simulink model "RNDBitGen"  (R2014b)
settings: Solver=FixedStepDiscrete  SolverMode=SingleTasking  StartTime=0.0  StopTime=20e-6*2  RelTol=1e-3
PreLoadFcn:
  | userName = getenv('UserName');
  | 
  | if strcmp(userName,'Tim')
  | cd C:\MA_1\RNDBitGen
  | else
  | cd D:\MA_1\RNDBitGen
  | end
InitFcn:
  | userName = getenv('UserName');
  | 
  | if strcmp(userName,'Tim')
  | cd C:\MA_1\RNDBitGen
  | else
  | cd D:\MA_1\RNDBitGen
  | end
libraries: xbsIndex_r4 x30
settings Model: Creator=Tim-UML  LastModifiedBy=Tim-UML
settings DebuggingCC: AssertControl=DisableAll
settings HardwareCC: ProdBitPerLong=64  ProdBitPerPointer=64  ProdWordSize=64  ProdHWDeviceType=Generic->64-bit Embedded Processor (LP64)  TargetHWDeviceType=32-bit Generic

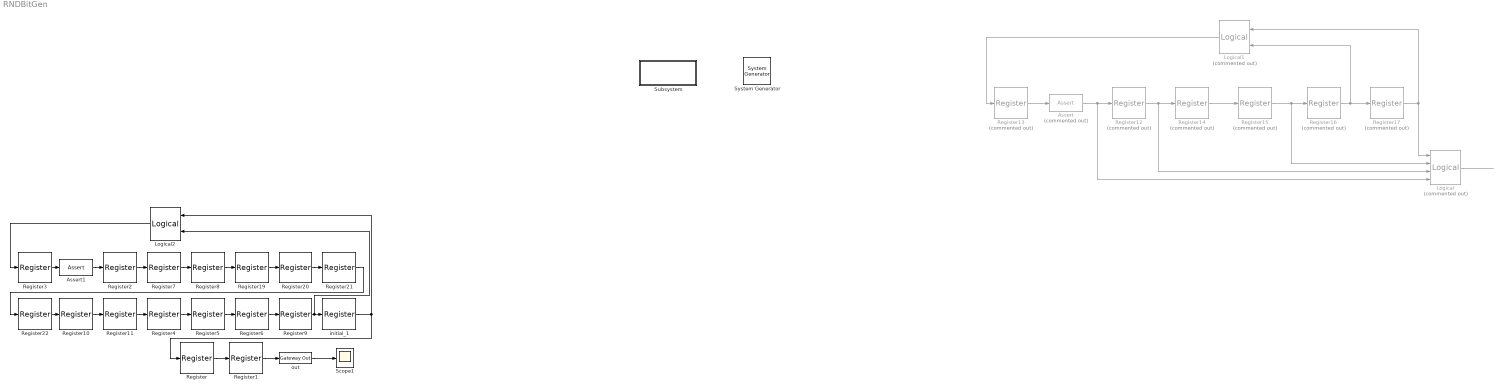
== system RNDBitGen ==
  " System Generator" : xbsIndex_r4/ System Generator  Tag=genX  xilinxfamily=zynq  part=xc7z020  speed=-1  package=clg400  synthesis_tool=Vivado  clock_wrapper=Clock Enables  directory=./netlistFin1  proj_type=Vivado  Synth_file=Vivado Synthesis Defaults  Impl_file=Vivado Implementation Defaults  testbench=on  simulink_period=sysgenSystemPeriod  sysclk_period=1000/250  dcm_input_clock_period=10  incr_netlist=off  trim_vbits=Everywhere in SubSystem  dbl_ovrd=According to Block Masks  core_generation=According to Block Masks  run_coregen=off  deprecated_control=off  eval_field=0  block_type=sysgen
  Assert : xbsIndex_r4/Assert  Commented=on  assert_type=on  type_source=Explicitly  gui_display_data_type=Boolean  arith_type=Boolean  n_bits=16  bin_pt=14  preci_type=Single  exp_width=8  frac_width=24  assert_rate=on  rate_source=Explicitly  period=Tb  output_port=on  block_type=assert
  Assert1 : xbsIndex_r4/Assert  assert_type=on  type_source=Explicitly  gui_display_data_type=Boolean  arith_type=Boolean  n_bits=16  bin_pt=14  preci_type=Single  exp_width=8  frac_width=24  assert_rate=on  rate_source=Explicitly  period=Tb  output_port=on  block_type=assert
  Logical : xbsIndex_r4/Logical  Commented=on  logical_function=XOR  inputs=4  en=off  latency=0  precision=Full  arith_type=Unsigned  n_bits=16  bin_pt=0  align_bp=on  dbl_ovrd=off  block_type=logical
  Logical1 : xbsIndex_r4/Logical  Commented=on  logical_function=XOR  inputs=2  en=off  latency=0  precision=Full  arith_type=Unsigned  n_bits=16  bin_pt=0  align_bp=on  dbl_ovrd=off  block_type=logical
  Logical2 : xbsIndex_r4/Logical  logical_function=XOR  inputs=2  en=off  latency=0  precision=Full  arith_type=Unsigned  n_bits=16  bin_pt=0  align_bp=on  dbl_ovrd=off  block_type=logical
  Register{,1..11,19..22} (16 alike) : xbsIndex_r4/Register  init=0  rst=off  en=off  dbl_ovrd=off  block_type=register
  Register{12..16} (5 alike) : xbsIndex_r4/Register  Commented=on  init=0  rst=off  en=off  dbl_ovrd=off  block_type=register
  Register17 : xbsIndex_r4/Register  Commented=on  init=1  rst=off  en=off  dbl_ovrd=off  block_type=register
  Scope1 : Scope
      settings: TimeRange=1.102458307597285e-07  YMin=-0  YMax=2  SaveName=ScopeData92
  Subsystem : Subsystem  mask(Model Parameters){upsample=No, dmtOfdm=DMT, guardInterval=Yes, AWGN=No, channel=No, equalizer=No, SampleTime=20e-9, BitTime=20e-9, modu_mode=0, radio_precision=fixpoint, bitCount=16, fracLen=13, impulseResponse=No}
      mask prompts: upsample "Enable Upsampling"; dmtOfdm "Select FFT Inputorder"; guardInterval "Guard Interval"; SampleTime "Sample Time [s]"; BitTime "Bit Time"; modu_mode "Modulation Mode"; radio_precision "Select Precision"; bitCount "Bit Count"; fracLen "Fraction Length"; impulseResponse "Measure Impulse Response"
      mask init:
      | initScript
      mask TypeOptions upsample: No | Yes
      mask TypeOptions dmtOfdm: OFDM | DMT
      mask TypeOptions guardInterval: No | Yes
      mask TypeOptions AWGN: No | Yes
      mask TypeOptions channel: No | Yes
      mask TypeOptions equalizer: No | Yes
      mask TypeOptions radio_precision: double | fixpoint
      mask TypeOptions impulseResponse: No | Yes
      mask DialogControl Container3 Prompt: Only for Fixpoint
      mask Display: disp('Edit Model\n Parameters')
  initial_1 : xbsIndex_r4/Register  init=1  rst=off  en=off  dbl_ovrd=off  block_type=register
  out : xbsIndex_r4/Gateway Out  inherit_from_input=on  hdl_port=on  rows=1  columns=1  UseAsDAC=off  DACChannel='1'  interface=None  automatic_assignment=on  address_offset=hex2dec('00')  intf_description=''  timing_constraint=None  locs_specified=off  LOCs={}  io_standard={}  block_type=gatewayout
  wires:
  out/1 -> Scope1/1
  Register/1 -> Register1/1
  Register1/1 -> out/1
  Register2/1 -> Register7/1
  Register3/1 -> Assert1/1
  Register7/1 -> Register8/1
  Register9/1 -> Logical2/2, initial_1/1
  initial_1/1 -> Logical2/1, Register/1
  Logical2/1 -> Register3/1
  Register8/1 -> Register19/1
  Assert1/1 -> Register2/1
  Register19/1 -> Register20/1
  Register20/1 -> Register21/1
  Register21/1 -> Register22/1
  Register22/1 -> Register10/1
  Register10/1 -> Register11/1
  Register11/1 -> Register4/1
  Register4/1 -> Register5/1
  Register5/1 -> Register6/1
  Register6/1 -> Register9/1
  Register12/1 -> Logical/3, Register14/1
  Register13/1 -> Assert/1
  Register14/1 -> Register15/1
  Register16/1 -> Logical1/2, Register17/1
  Register17/1 -> Logical/1, Logical1/1
  Logical1/1 -> Register13/1
  Register15/1 -> Logical/2, Register16/1
  Assert/1 -> Logical/4, Register12/1
  Logical/1 -> ?

== system RNDBitGen/Subsystem ==
